simulink model "DLHnguoc_3DOF"  (R2016b)
settings: Solver=VariableStepAuto  StartTime=0.0  StopTime=10.0  RelTol=1e-3
settings Model: Creator=Dell  LastModifiedBy=ADMIN

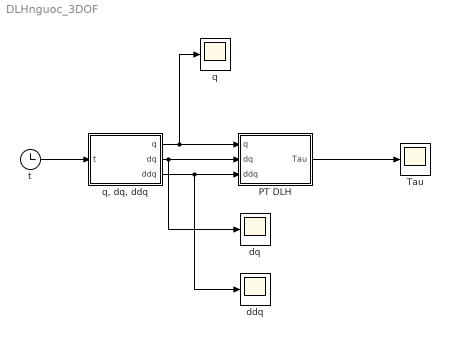
== system DLHnguoc_3DOF ==
  PT DLH : MATLAB Function  TreatAsAtomicUnit=on
  Tau : Scope
  ddq : Scope
  dq : Scope
  q : Scope
  "q, dq, ddq" : MATLAB Function  TreatAsAtomicUnit=on
  t : Clock
  wires:
  "q, dq, ddq"/1(q) -> q/1, PT DLH/1(q)
  t/1 -> "q, dq, ddq"/1(t)
  "q, dq, ddq"/2(dq) -> dq/1, PT DLH/2(dq)
  "q, dq, ddq"/3(ddq) -> ddq/1, PT DLH/3(ddq)
  PT DLH/1(Tau) -> Tau/1

== matlab function DLHnguoc_3DOF/PT DLH ==
  data: q input; Tau output; dq input; ddq input
function Tau=DLHN(q,dq,ddq)
[m1,m2,m3,L1,L2,L3,I1x,I1y,I1z,I2x,I2y,I2z,I3x,I3y,I3z]=parameter ();

% Khai bao ma tran khoi luong M
M=zeros(3,3);
M(1,1)= (9/4)*m1*L1^2+I1z+3*m2*L2*L1*cos(q(2))+L1^2*m2+(9/4)*m2*L2^2+I2y+2*m3*L2*L1*cos(q(2))+3*m3*L1*q(3)*sin(q(2))+L1^2*m3+L2^2*m3+(9/4)*m3*q(3)^2+I3y;
M(1,2)= (3/2)*m2*L2*L1*cos(q(2))+(9/4)*m2*L2^2+I2y+m3*L2*L1*cos(q(2))+(3/2)*m3*L1*q(3)*sin(q(2))+L2^2*m3+(9/4)*m3*q(3)^2+I3y;
M(1,3)= -(3/2)*L1*m3*cos(q(2))-(3/2)*L2*m3;


M(2,1)=(3/2)*m2*L2*L1*cos(q(2))+(9/4)*m2*L2^2+I2y+m3*L2*L1*cos(q(2))+(3/2)*m3*L1*q(3)*sin(q(2))+L2^2*m3+(9/4)*m3*q(3)^2+I3y;
M(2,2)=(9/4)*m2*L2^2+I2y+L2^2*m3+(9/4)*m3*q(3)^2+I3y;
M(2,3)=-(3/2)*L2*m3;

M(3,1)=-(3/2)*L1*m3*cos(q(2))-(3/2)*L2*m3;
M(3,2)=-(3/2)*L2*m3;
M(3,3)=(9/4)*m3;

% Khai bao ma tran Coriolis C
%h=-m2*L1*Lc2*sin(q(2));
Co=zeros(3,3);
Co(1,1)=-3*L1*L2*sin(q(2))*dq(2)*m2-2*L1*L2*sin(q(2))*dq(2)*m3+3*L1*cos(q(2))*dq(2)*m3*q(3)+3*L1*m3*sin(q(2))*dq(3)+(9/2)*m3*q(3)*dq(3);
Co(1,2)=-(3/2)*L1*L2*sin(q(2))*dq(2)*m2-L1*L2*sin(q(2))*dq(2)*m3+(3/2)*L1*cos(q(2))*dq(2)*m3*q(3)+(3/2)*L1*m3*sin(q(2))*dq(3)+(9/2)*m3*q(3)*dq(3);
Co(1,3)=(3/2)*L1*m3*sin(q(2))*dq(2);


Co(2,1)=(3/2)*L1*L2*sin(q(2))*dq(1)*m2+L1*L2*sin(q(2))*dq(1)*m3-(3/4)*L1*L2*sin(q(2))*dq(2)*m2-(1/2)*L1*L2*sin(q(2))*dq(2)*m3-(3/2)*L1*cos(q(2))*dq(1)*m3*q(3)+(3/4)*L1*cos(q(2))*dq(2)*m3*q(3)+(3/4)*L1*m3*sin(q(2))*dq(3)+(9/2)*m3*q(3)*dq(3);
Co(2,2)=(3/4)*L1*L2*sin(q(2))*dq(1)*m2+(1/2)*L1*L2*sin(q(2))*dq(1)*m3-(3/4)*L1*cos(q(2))*dq(1)*m3*q(3)+(9/2)*m3*q(3)*dq(3);
Co(2,3)=-(3/4)*L1*m3*sin(q(2))*dq(1);


Co(3,1)=-(3/2)*L1*m3*sin(q(2))*dq(1)+(3/4)*L1*m3*sin(q(2))*dq(2)-(9/4)*dq(1)*m3*q(3)-(9/4)*m3*q(3)*dq(2);
Co(3,2)=-(3/4)*L1*m3*sin(q(2))*dq(1)-(9/4)*dq(1)*m3*q(3)-(9/4)*m3*q(3)*dq(2);
Co(3,3)=0;

% Ma tran the nang hap dan
G=zeros(3,1);
G(1,1)=15*m1*L1*cos(q(1))+10*m2*L1*cos(q(1))+10*m3*L1*cos(q(1))+15*m2*L2*cos(q(1)+q(2))+10*m3*L2*cos(q(1)+q(2))+15*m3*sin(q(1)+q(2))*q(3);
G(2,1)=15*m2*L2*cos(q(1)+q(2))+10*m3*L2*cos(q(1)+q(2))+15*m3*sin(q(1)+q(2))*q(3);
G(3,1)=-15*m3*cos(q(1)+q(2));


% Pt DLH
Tau=M*ddq + Co*dq + G;

== matlab function DLHnguoc_3DOF/q, dq, ddq ==
  data: t input; q output; dq output; ddq output
function [q,dq,ddq] = fcn(t)
Pi=3.14;
q1 = (1/3)*Pi-(1/400)*t^2*Pi+(1/6000)*t^3*Pi;
q2 = (1/6)*Pi-(1/500)*t^2*Pi+(1/7500)*t^3*Pi;
q3 = 0.2-0.003*t^2+0.0002*t^3;

q=zeros(3,1);
q(1,1)=q1;
q(2,1)=q2;
q(3,1)=q3;

dq1=-(1/200)*t*Pi+(1/2000)*t^2*Pi;
dq2=-(1/250)*t*Pi+(1/2500)*t^2*Pi;
dq3=-0.006*t+0.0006*t^2;

dq=zeros(3,1);
dq(1,1)=dq1;
dq(2,1)=dq2;
dq(3,1)=dq3;

ddq1=-(1/200)*Pi+(1/1000)*t*Pi;
ddq2=-(1/250)*Pi+(1/1250)*t*Pi;
ddq3=-0.006+0.0012*t;

ddq=zeros(3,1);
ddq(1,1)=ddq1;
ddq(2,1)=ddq2;
ddq(3,1)=ddq3;
